simulink model "gentank"  (Simulink 6.4)
settings: Solver=ode45  StartTime=0.0  StopTime=10.0  RelTol=1e-3
values from neighbouring files (symbols this model uses):
  Ap = in(i,1)    [pid_fctn.m]
  Tc = 0.1*Td    [pid_fctn.m]
  Td = in(i,2)    [pid_fctn.m]
  Ti = in(i,3)    [pid_fctn.m]
settings Model: LastModifiedBy=gkovacs

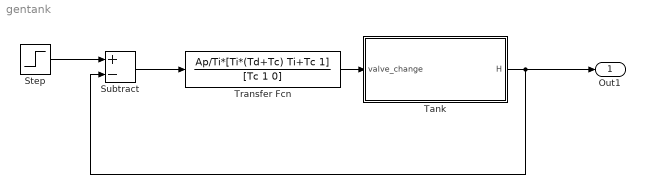
== system gentank ==
  Step : Step  SampleTime=0
  Subtract : Sum  Inputs=+-  OutScaling=2^-10
  Tank : Subsystem  mask(Tank){H_tank=2, A_tank=1, A_out=0.05, w_in-0.5=1}
      mask prompts: H_tank "Tank height"; A_tank "Tank area"; A_out "Cross-section of outflow pipe"; w_in-0.5 "Max inflow"
      mask help: Nonlinear model of free-outflow water tank with a valve on its input pipe.
      mask init:
      | H_tank=2;
      | A_tank=1;
      | A_out=0.05;
      | w_in=1;
  Transfer Fcn : TransferFcn  Numerator=Ap/Ti*[Ti*(Td+Tc) Ti+Tc 1]  Denominator=[Tc 1 0]
  Out1 : Outport
  wires:
  Transfer Fcn/1 -> Tank/1(valve_change)
  Subtract/1 -> Transfer Fcn/1
  Tank/1(H) -> Subtract/2, Out1/1
  Step/1 -> Subtract/1

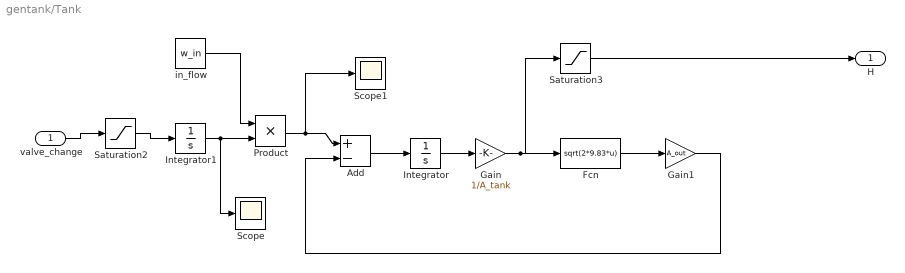
== system gentank/Tank ==
  valve_change : Inport
  Add : Sum  Inputs=+-  OutScaling=2^-10
  Fcn : Fcn  Expr=sqrt(2*9.83*u)
  Gain : Gain  Gain=1/A_tank
  Gain1 : Gain  Gain=A_out
  Integrator : Integrator
  Integrator1 : Integrator  LimitOutput=on  UpperSaturationLimit=1  LowerSaturationLimit=0
  Product : Product  RndMeth=Zero
  Saturation2 : Saturate  UpperLimit=5  LowerLimit=-5
  Saturation3 : Saturate  UpperLimit=H_tank  LowerLimit=0
  Scope : Scope
      settings: TimeRange=100  YMin=0  YMax=2  SaveName=ScopeData3
  Scope1 : Scope
      settings: TimeRange=100  YMin=0  YMax=2  SaveName=ScopeData4
  in_flow : Constant  Value=w_in  OutDataType=sfix(16)  ConRadixGroup=Use specified scaling  OutScaling=2^0  SampleTime=inf  FramePeriod=inf
  H : Outport
  wires:
  Add/1 -> Integrator/1
  Integrator/1 -> Gain/1
  Fcn/1 -> Gain1/1
  Gain1/1 -> Add/2
  in_flow/1 -> Product/1
  Integrator1/1 -> Product/2, Scope/1
  Product/1 -> Add/1, Scope1/1
  valve_change/1 -> Saturation2/1
  Saturation2/1 -> Integrator1/1
  Gain/1 -> Fcn/1, Saturation3/1
  Saturation3/1 -> H/1
